simulink model "q3"  (R2020b)
settings: Solver=VariableStepAuto  StartTime=0.0  StopTime=10.0  RelTol=1e-3
settings Model: Creator=Ravi  LastModifiedBy=Ravi

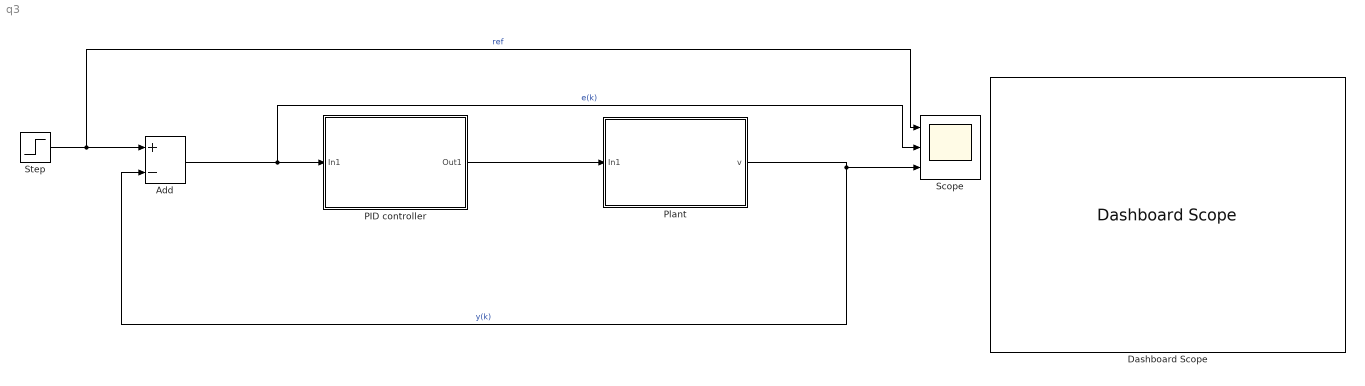
== system q3 ==
  Add : Sum  Inputs=+-
  Dashboard Scope : DashboardScope
  PID controller : Subsystem
  Plant : Subsystem
  Scope : Scope  NumInputPorts=3
  Step : Step  SampleTime=0
  wires:
  PID controller/1(Out1) -> Plant/1(In1)
  Plant/1(v) -> Scope/3, Add/2  "y(k)"
  Step/1 -> Scope/1, Add/1  "ref"
  Add/1 -> Scope/2, PID controller/1(In1)  "e(k)"

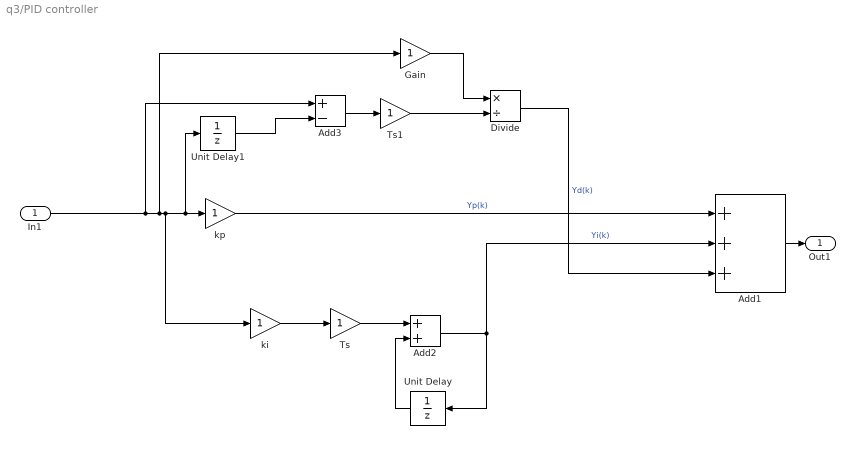
== system q3/PID controller ==
  In1 : Inport
  Add1 : Sum  Inputs=+++
  Add2 : Sum
  Add3 : Sum  Inputs=+-
  Divide : Product  Inputs=*/
  Gain : Gain
  Ts : Gain
  Ts1 : Gain
  Unit Delay : UnitDelay  SampleTime=-1  HasFrameUpgradeWarning=on
  Unit Delay1 : UnitDelay  SampleTime=-1  HasFrameUpgradeWarning=on
  ki : Gain
  kp : Gain
  Out1 : Outport
  wires:
  Add3/1 -> Ts1/1
  Ts/1 -> Add2/1
  Ts1/1 -> Divide/2
  Divide/1 -> Add1/3  "Yd(k)"
  Unit Delay1/1 -> Add3/2
  ki/1 -> Ts/1
  In1/1 -> Add3/1, Gain/1, ki/1, Unit Delay1/1, kp/1
  kp/1 -> Add1/1  "Yp(k)"
  Unit Delay/1 -> Add2/2
  Gain/1 -> Divide/1
  Add2/1 -> Unit Delay/1, Add1/2  "Yi(k)"
  Add1/1 -> Out1/1

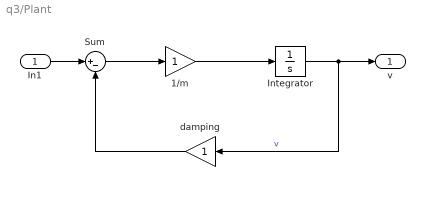
== system q3/Plant ==
  In1 : Inport
  1/m : Gain
  Integrator : Integrator
  Sum : Sum  Inputs=|+-
  damping : Gain
  v : Outport
  wires:
  Integrator/1 -> v/1, damping/1  "v"
  Sum/1 -> 1/m/1
  In1/1 -> Sum/1
  1/m/1 -> Integrator/1
  damping/1 -> Sum/2
